simulink model "Boost_Simplified_Model"  (R2024b)
settings: Solver=VariableStepAuto  StartTime=0.0  StopTime=10.0  MaxStep=1e-4  RelTol=1e-9
values from neighbouring files (symbols this model uses):
  C = .07e-3    (= 7e-05)    [Parameters.m]    (also in prelim.m)
  L = .3e-3    (= 0.0003)    [Parameters.m]    (also in prelim.m)
settings Model: Creator=jkord  LastModifiedBy=Αναστασία Λίβα

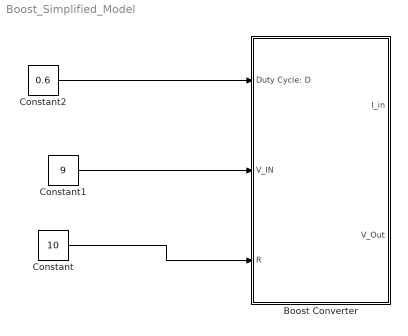
== system Boost_Simplified_Model ==
  Boost Converter : Subsystem
  Constant : Constant  Value=10
  Constant1 : Constant  Value=9
  Constant2 : Constant  Value=0.6
  wires:
  Constant/1 -> Boost Converter/3(R)
  Constant1/1 -> Boost Converter/2(V_IN)
  Constant2/1 -> Boost Converter/1(Duty Cycle: D)

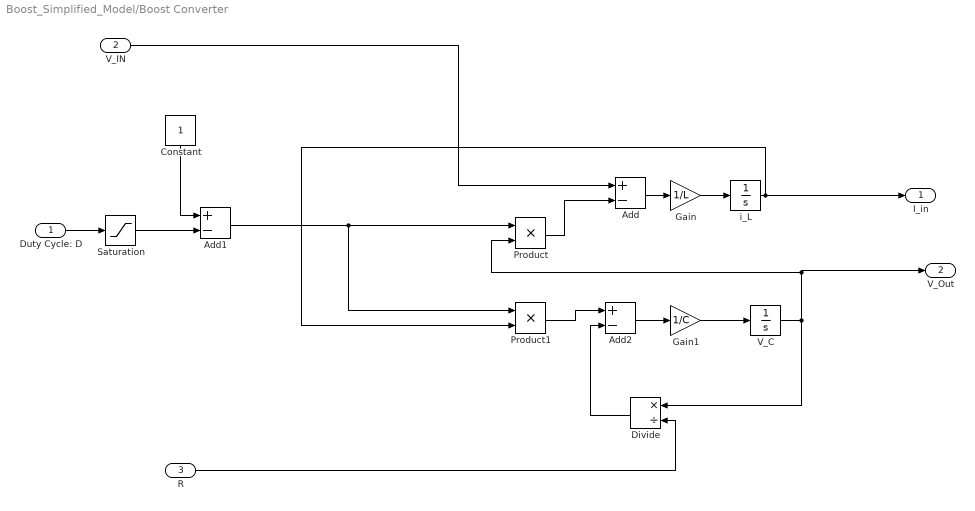
== system Boost_Simplified_Model/Boost Converter ==
  Duty Cycle: D : Inport
  V_IN : Inport  Port=2
  R : Inport  Port=3
  Add : Sum  Inputs=+-
  Add1 : Sum  Inputs=+-
  Add2 : Sum  Inputs=+-
  Constant : Constant
  Divide : Product  Inputs=*/
  Gain : Gain  Gain=1/L
  Gain1 : Gain  Gain=1/C
  Product : Product
  Product1 : Product
  Saturation : Saturate  UpperLimit=0.9  LowerLimit=0.1
  V_C : Integrator  InitialCondition=10
  i_L : Integrator  InitialCondition=2
  I_in : Outport
  V_Out : Outport  Port=2
  wires:
  Product/1 -> Add/2
  i_L/1 -> I_in/1, Product1/2
  Gain1/1 -> V_C/1
  V_IN/1 -> Add/1
  Gain/1 -> i_L/1
  V_C/1 -> Divide/1, V_Out/1, Product/2
  Add/1 -> Gain/1
  Product1/1 -> Add2/1
  Add2/1 -> Gain1/1
  Divide/1 -> Add2/2
  R/1 -> Divide/2
  Duty Cycle: D/1 -> Saturation/1
  Saturation/1 -> Add1/2
  Constant/1 -> Add1/1
  Add1/1 -> Product1/1, Product/1
